simulink model "simulink_model"  (R2018b)
settings: Solver=FixedStepDiscrete  StartTime=0.0  StopTime=inf  FixedStep=.001  RelTol=1e-3
libraries: LibrarySimulinkSAS x2, aerolibanimutils x1
settings Model: Creator=dds  LastModifiedBy=dds

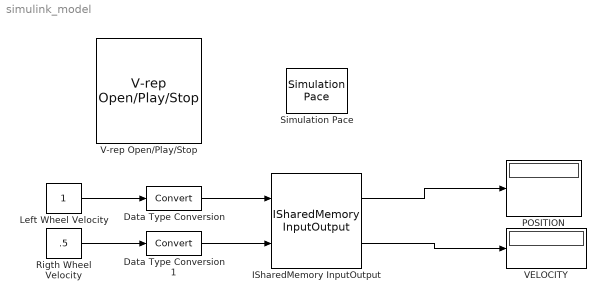
== system simulink_model ==
  Data Type Conversion : DataTypeConversion
  Data Type Conversion1 : DataTypeConversion
  ISharedMemory InputOutput : LibrarySimulinkSAS/ISharedMemory InputOutput  nameIn='wheel_velocity'  nameOut='position_velocity'  vecE=[1 1]  vecS=[3 2]  tipoE=['f' 'f']  tipoS=['f' 'f']  inOff=0  outOff=0  ts=-1  trigg=off
      settings: SourceProductName=Library SAS
  Left Wheel Velocity : Constant
  POSITION : Display
  Rigth Wheel Velocity : Constant  Value=.5
  Simulation Pace : aerolibanimutils/Simulation Pace  SimulationPace=1  SleepMode=Auto  OutputPaceError=off  SampleTime=-1
  V-rep Open/Play/Stop : LibrarySimulinkSAS/V-rep Open//Play//Stop  scene='scene.ttt'
      settings: SourceProductName=Library SAS
  VELOCITY : Display
  wires:
  Left Wheel Velocity/1 -> Data Type Conversion/1
  ISharedMemory InputOutput/1 -> POSITION/1
  ISharedMemory InputOutput/2 -> VELOCITY/1
  Data Type Conversion/1 -> ISharedMemory InputOutput/1
  Data Type Conversion1/1 -> ISharedMemory InputOutput/2
  Rigth Wheel Velocity/1 -> Data Type Conversion1/1
